simulink model "jianmo_2"  (R2020b)
settings: Solver=VariableStepAuto  StartTime=0.0  StopTime=100  RelTol=1e-3
settings Model: Creator=19017  LastModifiedBy=19017

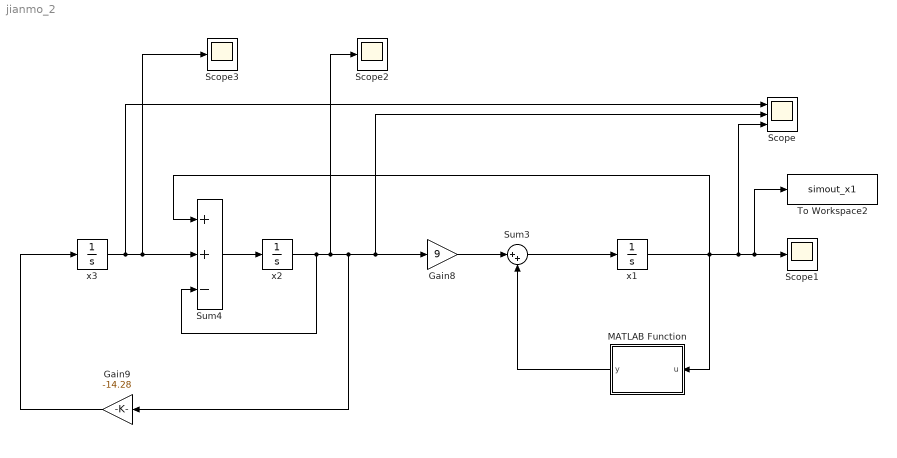
== system jianmo_2 ==
  Gain8 : Gain  Gain=9
  Gain9 : Gain  Gain=-14.28
  MATLAB Function : MATLAB Function  TreatAsAtomicUnit=on
  Scope : Scope  NumInputPorts=3
  Scope1 : Scope
  Scope2 : Scope
  Scope3 : Scope
  Sum3 : Sum  Inputs=|++
  Sum4 : Sum  Inputs=++-
  To Workspace2 : ToWorkspace  VariableName=simout_x1  SaveFormat=Timeseries  SampleTime=-1
  x1 : Integrator  InitialCondition=-0.1
  x2 : Integrator  InitialCondition=0.1
  x3 : Integrator  InitialCondition=0.2
  wires:
  x3/1 -> Scope/1, Scope3/1, Sum4/2
  MATLAB Function/1(y) -> Sum3/2
  Gain9/1 -> x3/1
  Gain8/1 -> Sum3/1
  Sum4/1 -> x2/1
  x1/1 -> MATLAB Function/1(u), Scope/3, To Workspace2/1, Scope1/1, Sum4/1
  Sum3/1 -> x1/1
  x2/1 -> Sum4/3, Scope2/1, Gain9/1, Scope/2, Gain8/1

== matlab function jianmo_2/MATLAB Function ==
  data: u input; y output
function y = fcn(u)
x1=u;
x1dao=-((2*9)/7)*x1+(((9*3)/7)/2)*(abs(x1+1)-abs(x1-1))
y=x1dao;
